simulink model "Electrothermal_Battery_v2_Simulation_Feedback"  (R2021a)
settings: Solver=FixedStepAuto  StartTime=0.0  StopTime=t  FixedStep=dt  RelTol=1e-3  EnableMultiTasking=on
undefined symbols (not defined in the file or in its folder): Ion, Li
libraries: simulink x4, Lib_EMTAT x2
settings Model: Creator=ewong  LastModifiedBy=mebell
settings SolverCC: AlgebraicLoopSolver=LineSearch
settings DataIOCC: ReturnWorkspaceOutputs=off
settings OptimizationCC: LifeSpan=inf
settings DebuggingCC: PregeneratedLibrarySubsystemCodeDiagnostic=none  SFUnexpectedBacktrackingDiag=warning  SFNoUnconditionalDefaultTransitionDiag=warning  SFExecutionAtInitializationDiag=none  SFMachineParentedDataDiag=warning  ArithmeticOperatorsInVariantConditions=warning
settings SFSimCC: SimUseLocalCustomCode=off  CustomCodeUndefinedFunction=UseInterfaceOnly
settings RTWCC: RTWUseLocalCustomCode=off
settings CodeAppCC: StateflowObjectComments=on
settings GRTTargetCC: TargetLangStandard=C89/C90 (ANSI)
settings ConfigComp: CovMetricSettings=dw  CovSaveCumulativeToWorkspaceVar=on  CovSaveSingleToWorkspaceVar=on  CovExternalEMLEnable=off

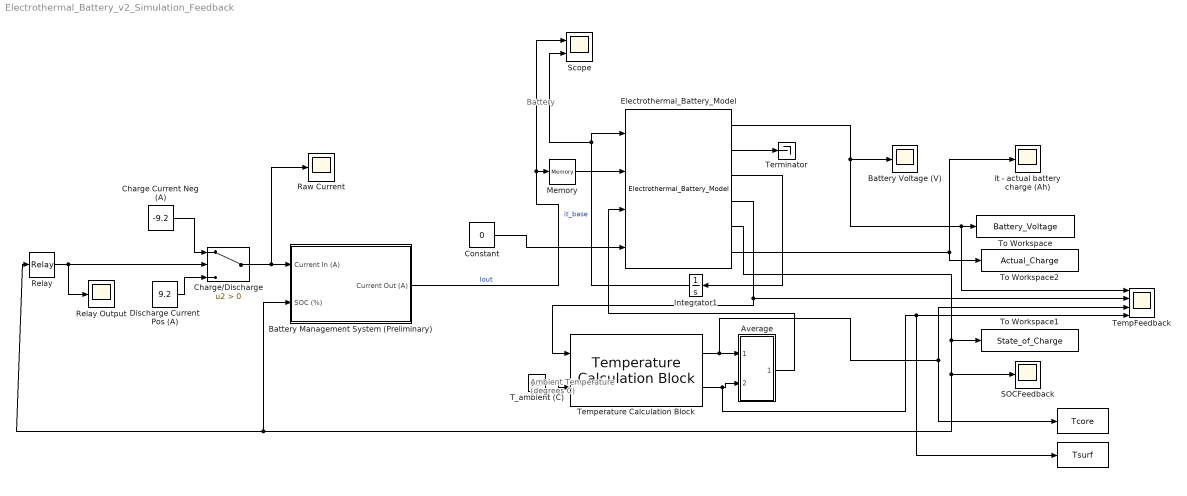
== system Electrothermal_Battery_v2_Simulation_Feedback ==
  note: Battery
  note: Ambient Temperature
      | (degrees C)
  " " : ToWorkspace  VariableName=Tsurf  SampleTime=-1
  "  " : ToWorkspace  VariableName=Tcore  SampleTime=-1
  Average : Subsystem
  Battery Management System (Preliminary) : Subsystem
  Battery Voltage (V) : Scope
  Charge Current Neg (A) : Constant  Value=-9.2
  Charge/Discharge : Switch  Criteria=u2 > Threshold
  Constant : Constant  Value=0
  Discharge Current Pos (A) : Constant  Value=9.2
  Electrothermal_Battery_Model : Lib_EMTAT/Components/Physics-Based/Electrothermal_Battery_Model  E0_M=E0_M  Q_M=Q_M  R_M=R_M  K_M=K_M  B_M=B_M  SOC_Init_M=SOC_Init_M  A_M=A_M  battery_type_M=Li-Ion  TempIn=Celsius  BWS=on  thermal=on  nameField=Thermal Model
      settings: SourceProductName=EMTAT
  Integrator1 : Integrator
  Memory : Memory
  Raw Current : Scope
  Relay : Relay  OnSwitchValue=99  OffSwitchValue=3  OnOutputValue=0  OffOutputValue=5
  Relay Output : Scope
  SOCFeedback : Scope
  Scope : Scope  NumInputPorts=2
  T_ambient (C) : Constant  Value=528
  TempFeedback : Scope  NumInputPorts=4
  Temperature Calculation Block : Lib_EMTAT/Components/Physics-Based/Temperature Calculation Block  Tj_0_M=25  Ts_0_M=25  Cj_M=Cj  Rj_M=Rj  Ru_M=Ru  Cs_M=Cs
      settings: SourceProductName=EMTAT
  Terminator : Terminator
  To Workspace : ToWorkspace  VariableName=Battery_Voltage  SampleTime=-1
  To Workspace1 : ToWorkspace  VariableName=State_of_Charge  SampleTime=-1
  To Workspace2 : ToWorkspace  VariableName=Actual_Charge  SampleTime=-1
  it - actual battery charge (Ah) : Scope
  wires:
  Discharge Current Pos (A)/1 -> Charge/Discharge/3
  Charge Current Neg (A)/1 -> Charge/Discharge/1
  Relay/1 -> Relay Output/1, Charge/Discharge/2
  Electrothermal_Battery_Model/5 -> Battery Management System (Preliminary)/2(SOC (%)), Relay/1, SOCFeedback/1, To Workspace1/1
  Charge/Discharge/1 -> Raw Current/1, Battery Management System (Preliminary)/1(Current In (A))
  Electrothermal_Battery_Model/6 -> To Workspace2/1, it - actual battery charge (Ah)/1
  Temperature Calculation Block/1 -> TempFeedback/3, "  "/1, Average/1(In1)
  Temperature Calculation Block/2 -> TempFeedback/4, " "/1, Average/2(In2)
  Electrothermal_Battery_Model/4 -> Temperature Calculation Block/1, TempFeedback/2
  Electrothermal_Battery_Model/3 -> Integrator1/1
  Integrator1/1 -> Electrothermal_Battery_Model/1, Scope/2  "it_base"
  Average/1(Out1) -> Electrothermal_Battery_Model/3
  Battery Management System (Preliminary)/1(Current Out (A)) -> Scope/1, Memory/1  "Iout"
  Electrothermal_Battery_Model/1 -> TempFeedback/1, To Workspace/1, Battery Voltage (V)/1
  T_ambient (C)/1 -> Temperature Calculation Block/2
  Memory/1 -> Electrothermal_Battery_Model/2
  Electrothermal_Battery_Model/2 -> Terminator/1
  Constant/1 -> Electrothermal_Battery_Model/4

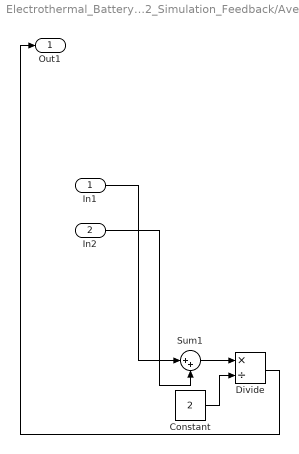
== system Electrothermal_Battery_v2_Simulation_Feedback/Average ==
  In1 : Inport
  In2 : Inport  Port=2
  Constant : Constant  Value=2
  Divide : Product  Inputs=*/
  Sum1 : Sum  Inputs=|++
  Out1 : Outport  VectorParamsAs1DForOutWhenUnconnected=off
  wires:
  In1/1 -> Sum1/1
  Sum1/1 -> Divide/1
  In2/1 -> Sum1/2
  Constant/1 -> Divide/2
  Divide/1 -> Out1/1

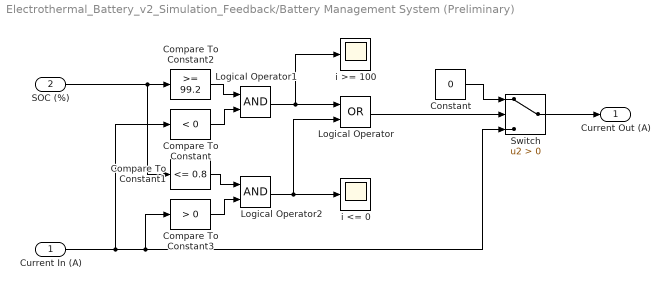
== system Electrothermal_Battery_v2_Simulation_Feedback/Battery Management System (Preliminary) ==
  Current In (A) : Inport
  SOC (%) : Inport  Port=2
  Compare To Constant : simulink/Logic and Bit Operations/Compare To Constant  relop=<  const=0  OutDataTypeStr=boolean
  Compare To Constant1 : simulink/Logic and Bit Operations/Compare To Constant  relop=<=  const=0.8  OutDataTypeStr=boolean
  Compare To Constant2 : simulink/Logic and Bit Operations/Compare To Constant  relop=>=  const=99.2  OutDataTypeStr=boolean
  Compare To Constant3 : simulink/Logic and Bit Operations/Compare To Constant  relop=>  const=0  OutDataTypeStr=boolean
  Constant : Constant  Value=0
  Logical Operator : Logic  Operator=OR  AllPortsSameDT=off  OutDataTypeStr=boolean
  Logical Operator1 : Logic  AllPortsSameDT=off  OutDataTypeStr=boolean
  Logical Operator2 : Logic  AllPortsSameDT=off  OutDataTypeStr=boolean
  Switch : Switch  Criteria=u2 > Threshold
  i <= 0 : Scope
  i >= 100 : Scope
  Current Out (A) : Outport  VectorParamsAs1DForOutWhenUnconnected=off
  wires:
  Constant/1 -> Switch/1
  Logical Operator/1 -> Switch/2
  Current In (A)/1 -> Compare To Constant/1, Compare To Constant3/1, Switch/3
  SOC (%)/1 -> Compare To Constant1/1, Compare To Constant2/1
  Compare To Constant2/1 -> Logical Operator1/1
  Compare To Constant/1 -> Logical Operator1/2
  Compare To Constant1/1 -> Logical Operator2/1
  Compare To Constant3/1 -> Logical Operator2/2
  Logical Operator1/1 -> i >= 100/1, Logical Operator/1
  Logical Operator2/1 -> i <= 0/1, Logical Operator/2
  Switch/1 -> Current Out (A)/1
